simulink model "controllo_disco_rigido_ritardo"  (R2019b)
settings: Solver=VariableStepAuto  StartTime=0.0  StopTime=5  FixedStep=0.01  RelTol=1e-3
values from neighbouring files (symbols this model uses):
  b = 0.002    [controllo_disco_rigido.m]    (also in controllo_disco_rigido_baseWS.mat; controllo_disco_rigido_script.m; init_controllo_disco_rigido.m)
  delay = 0.3    [controllo_disco_rigido.m]    (also in controllo_disco_rigido_script.m)
  J = 0.001    [controllo_disco_rigido.m]    (also in controllo_disco_rigido_baseWS.mat; controllo_disco_rigido_script.m; init_controllo_disco_rigido.m)
  k = (1/67.5)*gsys(3)    [controllo_disco_rigido_script.m]
  R1_n = 35000    [controllo_disco_rigido_script.m]
  R2_pole_n = [-500, -1400]    [controllo_disco_rigido_script.m]
  R2_zero_n = [-2]    [controllo_disco_rigido_script.m]
  ritardo = exp(-delay*s)    [controllo_disco_rigido_script.m]
  W_pole = max(R2_pole_n)    [controllo_disco_rigido_script.m]
  y0 = 300    [controllo_disco_rigido.m]    (also in controllo_disco_rigido_script.m)
libraries: cstblocks x2
settings Model: Creator=Utente  LastModifiedBy=Utente
settings DataIOCC: ReturnWorkspaceOutputsName=MdlFnl

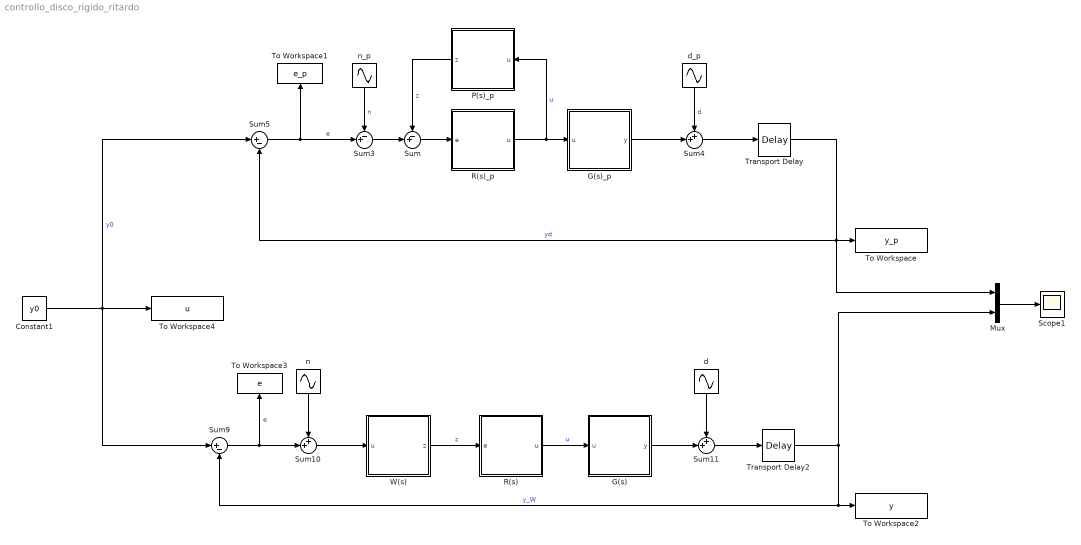
== system controllo_disco_rigido_ritardo ==
  Constant1 : Constant  Value=y0
  G(s) : Subsystem
  G(s)_p : Subsystem
  Mux : Mux  Inputs=2
  P(s)_p : Subsystem
  R(s) : Subsystem
  R(s)_p : Subsystem
  Scope1 : Scope
  Sum : Sum  Inputs=-+|
  Sum10 : Sum  Inputs=++|
  Sum11 : Sum  Inputs=++|
  Sum3 : Sum  Inputs=-+|
  Sum4 : Sum  Inputs=++|
  Sum5 : Sum  Inputs=|+-
  Sum9 : Sum  Inputs=|+-
  To Workspace : ToWorkspace  VariableName=y_p  SampleTime=-1
  To Workspace1 : ToWorkspace  VariableName=e_p  SampleTime=-1
  To Workspace2 : ToWorkspace  VariableName=y  SampleTime=-1
  To Workspace3 : ToWorkspace  VariableName=e  SampleTime=-1
  To Workspace4 : ToWorkspace  VariableName=u  SampleTime=-1
  Transport Delay : TransportDelay  DelayTime=delay
  Transport Delay2 : TransportDelay  DelayTime=delay
  W(s) : Subsystem
  d : Sin  Frequency=[5]  SampleTime=0
  d_p : Sin  Frequency=[5]  SampleTime=0
  n : Sin  Frequency=[50]  SampleTime=0
  n_p : Sin  Frequency=[50]  SampleTime=0
  wires:
  n_p/1 -> Sum3/1  "n"
  Sum5/1 -> Sum3/2, To Workspace1/1  "e"
  d_p/1 -> Sum4/1  "d"
  Constant1/1 -> Sum5/1, To Workspace4/1, Sum9/1  "y0"
  R(s)_p/1(u) -> P(s)_p/1(u), G(s)_p/1(u)  "u"
  G(s)_p/1(y) -> Sum4/2
  Sum4/1 -> Transport Delay/1
  Transport Delay/1 -> Mux/1, To Workspace/1, Sum5/2  "yd"
  Sum/1 -> R(s)_p/1(e)
  Sum3/1 -> Sum/2
  P(s)_p/1(z) -> Sum/1  "z"
  Sum11/1 -> Transport Delay2/1
  Transport Delay2/1 -> Mux/2, Sum9/2, To Workspace2/1  "y_W"
  n/1 -> Sum10/1
  G(s)/1(y) -> Sum11/2
  d/1 -> Sum11/1
  W(s)/1(z) -> R(s)/1(e)  "z"
  Sum10/1 -> W(s)/1(u)
  R(s)/1(u) -> G(s)/1(u)  "u"
  Mux/1 -> Scope1/1
  Sum9/1 -> Sum10/2, To Workspace3/1  "e"

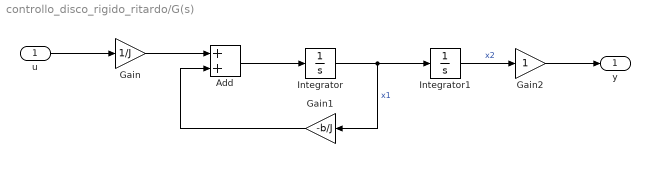
== system controllo_disco_rigido_ritardo/G(s) ==
  u : Inport
  Add : Sum
  Gain : Gain  Gain=1/J
  Gain1 : Gain  Gain=-b/J
  Gain2 : Gain
  Integrator : Integrator
  Integrator1 : Integrator
  y : Outport
  wires:
  Integrator/1 -> Gain1/1, Integrator1/1  "x1"
  u/1 -> Gain/1
  Add/1 -> Integrator/1
  Gain/1 -> Add/1
  Gain1/1 -> Add/2
  Integrator1/1 -> Gain2/1  "x2"
  Gain2/1 -> y/1

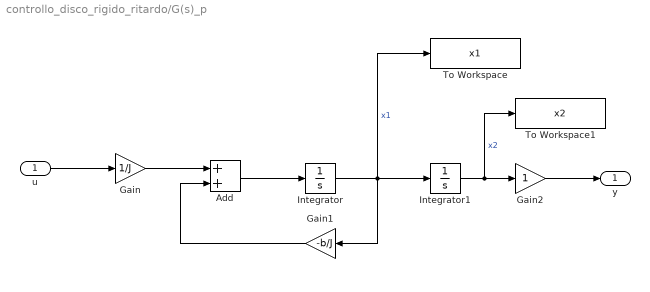
== system controllo_disco_rigido_ritardo/G(s)_p ==
  u : Inport
  Add : Sum
  Gain : Gain  Gain=1/J
  Gain1 : Gain  Gain=-b/J
  Gain2 : Gain
  Integrator : Integrator
  Integrator1 : Integrator
  To Workspace : ToWorkspace  VariableName=x1  SampleTime=-1
  To Workspace1 : ToWorkspace  VariableName=x2  SampleTime=-1
  y : Outport
  wires:
  Integrator/1 -> To Workspace/1, Gain1/1, Integrator1/1  "x1"
  u/1 -> Gain/1
  Add/1 -> Integrator/1
  Gain/1 -> Add/1
  Gain1/1 -> Add/2
  Integrator1/1 -> Gain2/1, To Workspace1/1  "x2"
  Gain2/1 -> y/1

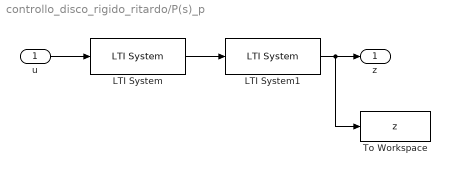
== system controllo_disco_rigido_ritardo/P(s)_p ==
  u : Inport
  LTI System : cstblocks/LTI System  sys=sys_tf  IC=[]
  LTI System1 : cstblocks/LTI System  sys=1-ritardo  IC=[]
  To Workspace : ToWorkspace  VariableName=z  SampleTime=-1
  z : Outport
  wires:
  u/1 -> LTI System/1
  LTI System1/1 -> To Workspace/1, z/1
  LTI System/1 -> LTI System1/1

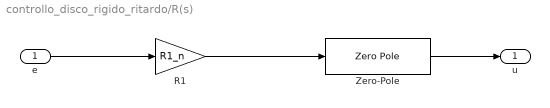
== system controllo_disco_rigido_ritardo/R(s) ==
  e : Inport
  R1 : Gain  Gain=R1_n
  Zero-Pole : ZeroPole  Zeros=R2_zero_n  Poles=R2_pole_n
  u : Outport
  wires:
  e/1 -> R1/1
  R1/1 -> Zero-Pole/1
  Zero-Pole/1 -> u/1

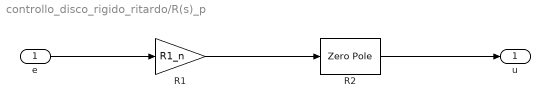
== system controllo_disco_rigido_ritardo/R(s)_p ==
  e : Inport
  R1 : Gain  Gain=R1_n
  R2 : ZeroPole  Zeros=R2_zero_n  Poles=R2_pole_n
  u : Outport
  wires:
  R1/1 -> R2/1
  e/1 -> R1/1
  R2/1 -> u/1

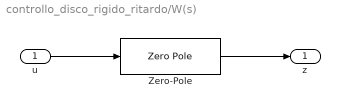
== system controllo_disco_rigido_ritardo/W(s) ==
  u : Inport
  Zero-Pole : ZeroPole  Zeros=[]  Poles=W_pole  Gain=k
  z : Outport
  wires:
  u/1 -> Zero-Pole/1
  Zero-Pole/1 -> z/1
